simulink model "PID_conroller"  (R2020b)
settings: Solver=VariableStepAuto  StartTime=0.0  StopTime=120  RelTol=1e-3
PreLoadFcn:
  | clear all;
  | close all;
  | clc;
  | m=1000;
  | b=50;
  | u=500;
settings Model: DataDictionary=data_dictionary.sldd  Creator=Aradhana desai  LastModifiedBy=Aradhana desai
settings DataIOCC: SaveOutput=off  SaveTime=off

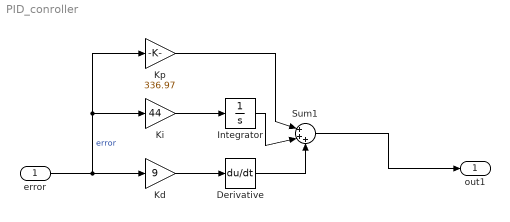
== system PID_conroller ==
  error : Inport  OutDataTypeStr=double  PortDimensions=1  SampleTime=0
  Derivative : Derivative
  Integrator : Integrator
  Kd : Gain  Gain=9
  Ki : Gain  Gain=44
  Kp : Gain  Gain=336.97
  Sum1 : Sum  Inputs=|+++
  out1 : Outport  OutDataTypeStr=double  PortDimensions=1  SampleTime=0
  wires:
  Kd/1 -> Derivative/1
  Ki/1 -> Integrator/1
  error/1 -> Kp/1, Ki/1, Kd/1  "error"
  Derivative/1 -> Sum1/3
  Sum1/1 -> out1/1
  Kp/1 -> Sum1/1
  Integrator/1 -> Sum1/2
